simulink model "DAQTest"  (Simulink 7.9)
settings: Solver=FixedStepDiscrete  StartTime=0.0  StopTime=inf  FixedStep=0.001  RelTol=1e-3
undefined symbols (not defined in the file or in its folder): CalibrationParams, EncoderAngleLimits, EncoderThreshold, IMUAngleLimits, IMUThreshold, MotorParams
libraries: xpcethercatlib x160, simulink x3, marlo_lib_v01 x2, dspswit3 x1
(part 1 of 3)
settings Model: Creator=bgbuss  LastModifiedBy=bgbuss  BufferReuse=off
settings DataIOCC: LimitDataPoints=off
settings OptimizationCC: BlockReduction=off  OptimizeBlockIOStorage=off  BufferReuse=off  ExpressionFolding=off  LocalBlockOutputs=off
settings HardwareCC: ProdIntDivRoundTo=Zero  ProdEndianess=LittleEndian  ProdHWDeviceType=Generic->32-bit x86 compatible
settings RTWCC: SystemTargetFile=xpctarget.tlc  TemplateMakefile=xpc_default_tmf  Description=xPC Target  ProcessScript=xpctarget_make_rtw_hook  RTWCompilerOptimization=On
settings xpcTargetCC: TargetFcnLib=ansi_tfl_table_tmw.mat  CodeReplacementLibrary=XPC_BLAS  CodeExecutionProfiling=off  ParMdlRefBuildCompliant=on  ConcurrentExecutionCompliant=on  CombineSignalStateStructs=off  PortableWordSizes=off  GRTInterface=on  RL32LogBufSizeModifier=20000000  xPCTaskExecutionProfile=off  xPCRL32EventNumber=5000  xPCLoadParamSetFile=off  xPCConcurrentTasks=off  xPCEnableSFAnimation=off

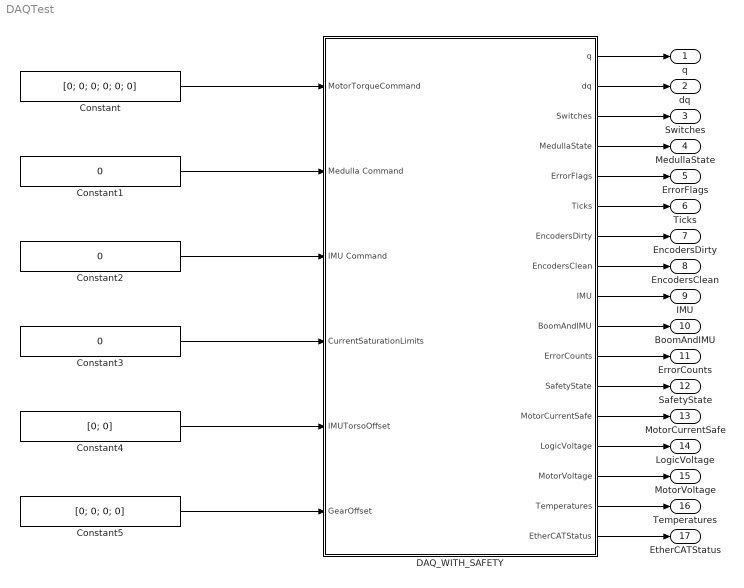
== system DAQTest ==
  Constant : Constant  Value=[0; 0; 0; 0; 0; 0]
  Constant1 : Constant  Value=0
  Constant2 : Constant  Value=0
  Constant3 : Constant  Value=0
  Constant4 : Constant  Value=[0; 0]
  Constant5 : Constant  Value=[0; 0; 0; 0]
  DAQ_WITH_SAFETY : Subsystem  AncestorBlock=marlo_lib_v01/DAQ_WITH_SAFETY
  q : Outport
  dq : Outport  Port=2
  Switches : Outport  Port=3
  MedullaState : Outport  Port=4
  ErrorFlags : Outport  Port=5
  Ticks : Outport  Port=6
  EncodersDirty : Outport  Port=7
  EncodersClean : Outport  Port=8
  IMU : Outport  Port=9
  BoomAndIMU : Outport  Port=10
  ErrorCounts : Outport  Port=11
  SafetyState : Outport  Port=12
  MotorCurrentSafe : Outport  Port=13
  LogicVoltage : Outport  Port=14
  MotorVoltage : Outport  Port=15
  Temperatures : Outport  Port=16
  EtherCATStatus : Outport  Port=17
  wires:
  DAQ_WITH_SAFETY/1(q) -> q/1
  DAQ_WITH_SAFETY/2(dq) -> dq/1
  DAQ_WITH_SAFETY/3(Switches) -> Switches/1
  DAQ_WITH_SAFETY/4(MedullaState) -> MedullaState/1
  DAQ_WITH_SAFETY/5(ErrorFlags) -> ErrorFlags/1
  DAQ_WITH_SAFETY/6(Ticks) -> Ticks/1
  DAQ_WITH_SAFETY/7(EncodersDirty) -> EncodersDirty/1
  DAQ_WITH_SAFETY/8(EncodersClean) -> EncodersClean/1
  DAQ_WITH_SAFETY/9(IMU) -> IMU/1
  DAQ_WITH_SAFETY/10(BoomAndIMU) -> BoomAndIMU/1
  DAQ_WITH_SAFETY/11(ErrorCounts) -> ErrorCounts/1
  DAQ_WITH_SAFETY/12(SafetyState) -> SafetyState/1
  DAQ_WITH_SAFETY/13(MotorCurrentSafe) -> MotorCurrentSafe/1
  Constant/1 -> DAQ_WITH_SAFETY/1(MotorTorqueCommand)
  Constant1/1 -> DAQ_WITH_SAFETY/2(Medulla Command)
  Constant2/1 -> DAQ_WITH_SAFETY/3(IMU Command)
  Constant3/1 -> DAQ_WITH_SAFETY/4(CurrentSaturationLimits)
  Constant4/1 -> DAQ_WITH_SAFETY/5(IMUTorsoOffset)
  Constant5/1 -> DAQ_WITH_SAFETY/6(GearOffset)
  DAQ_WITH_SAFETY/17(EtherCATStatus) -> EtherCATStatus/1
  DAQ_WITH_SAFETY/16(Temperatures) -> Temperatures/1
  DAQ_WITH_SAFETY/14(LogicVoltage) -> LogicVoltage/1
  DAQ_WITH_SAFETY/15(MotorVoltage) -> MotorVoltage/1

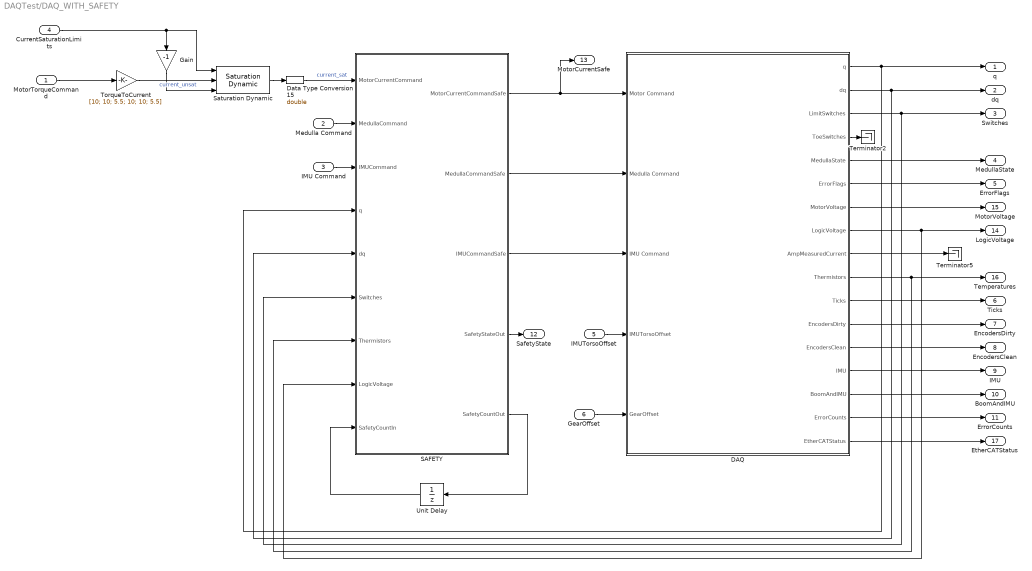
== system DAQTest/DAQ_WITH_SAFETY ==
  MotorTorqueCommand : Inport
  Medulla Command : Inport  Port=2
  IMU Command : Inport  Port=3
  CurrentSaturationLimits : Inport  Port=4
  IMUTorsoOffset : Inport  Port=5
  GearOffset : Inport  Port=6
  DAQ : Subsystem
  Data Type Conversion15 : DataTypeConversion  OutDataTypeStr=double
  Gain : Gain  Gain=-1
  SAFETY : MATLAB Function  TreatAsAtomicUnit=on
  Saturation Dynamic : simulink/Discontinuities/Saturation Dynamic  OutMin=[]  OutMax=[]  OutDataTypeStr=Inherit: Same as second input  OutDataType=fixdt(1, 16)  OutScaling=2^-10  DoSatur=off
  Terminator2 : Terminator
  Terminator5 : Terminator
  TorqueToCurrent : Gain  Gain=[10; 10; 5.5; 10; 10; 5.5]
  Unit Delay : UnitDelay  SampleTime=-1
  q : Outport
  dq : Outport  Port=2
  Switches : Outport  Port=3
  MedullaState : Outport  Port=4
  ErrorFlags : Outport  Port=5
  Ticks : Outport  Port=6
  EncodersDirty : Outport  Port=7
  EncodersClean : Outport  Port=8
  IMU : Outport  Port=9
  BoomAndIMU : Outport  Port=10
  ErrorCounts : Outport  Port=11
  SafetyState : Outport  Port=12
  MotorCurrentSafe : Outport  Port=13
  LogicVoltage : Outport  Port=14
  MotorVoltage : Outport  Port=15
  Temperatures : Outport  Port=16
  EtherCATStatus : Outport  Port=17
  wires:
  DAQ/13(EncodersClean) -> EncodersClean/1
  DAQ/16(ErrorCounts) -> ErrorCounts/1
  Unit Delay/1 -> SAFETY/9(SafetyCountIn)
  SAFETY/5(SafetyCountOut) -> Unit Delay/1
  GearOffset/1 -> DAQ/5(GearOffset)
  IMUTorsoOffset/1 -> DAQ/4(IMUTorsoOffset)
  DAQ/15(BoomAndIMU) -> BoomAndIMU/1
  Data Type Conversion15/1 -> SAFETY/1(MotorCurrentCommand)  "current_sat"
  SAFETY/2(MedullaCommandSafe) -> DAQ/2(Medulla Command)
  SAFETY/1(MotorCurrentCommandSafe) -> MotorCurrentSafe/1, DAQ/1(Motor Command)
  Gain/1 -> Saturation Dynamic/3
  CurrentSaturationLimits/1 -> Gain/1, Saturation Dynamic/1
  Saturation Dynamic/1 -> Data Type Conversion15/1
  DAQ/6(ErrorFlags) -> ErrorFlags/1
  DAQ/5(MedullaState) -> MedullaState/1
  DAQ/9(AmpMeasuredCurrent) -> Terminator5/1
  DAQ/7(MotorVoltage) -> MotorVoltage/1
  DAQ/10(Thermistors) -> SAFETY/7(Thermistors), Temperatures/1
  TorqueToCurrent/1 -> Saturation Dynamic/2  "current_unsat"
  SAFETY/4(SafetyStateOut) -> SafetyState/1
  DAQ/14(IMU) -> IMU/1
  DAQ/8(LogicVoltage) -> SAFETY/8(LogicVoltage), LogicVoltage/1
  DAQ/3(LimitSwitches) -> Switches/1, SAFETY/6(Switches)
  DAQ/2(dq) -> dq/1, SAFETY/5(dq)
  DAQ/1(q) -> q/1, SAFETY/4(q)
  IMU Command/1 -> SAFETY/3(IMUCommand)
  Medulla Command/1 -> SAFETY/2(MedullaCommand)
  MotorTorqueCommand/1 -> TorqueToCurrent/1
  SAFETY/3(IMUCommandSafe) -> DAQ/3(IMU Command)
  DAQ/11(Ticks) -> Ticks/1
  DAQ/12(EncodersDirty) -> EncodersDirty/1
  DAQ/4(ToeSwitches) -> Terminator2/1
  DAQ/17(EtherCATStatus) -> EtherCATStatus/1

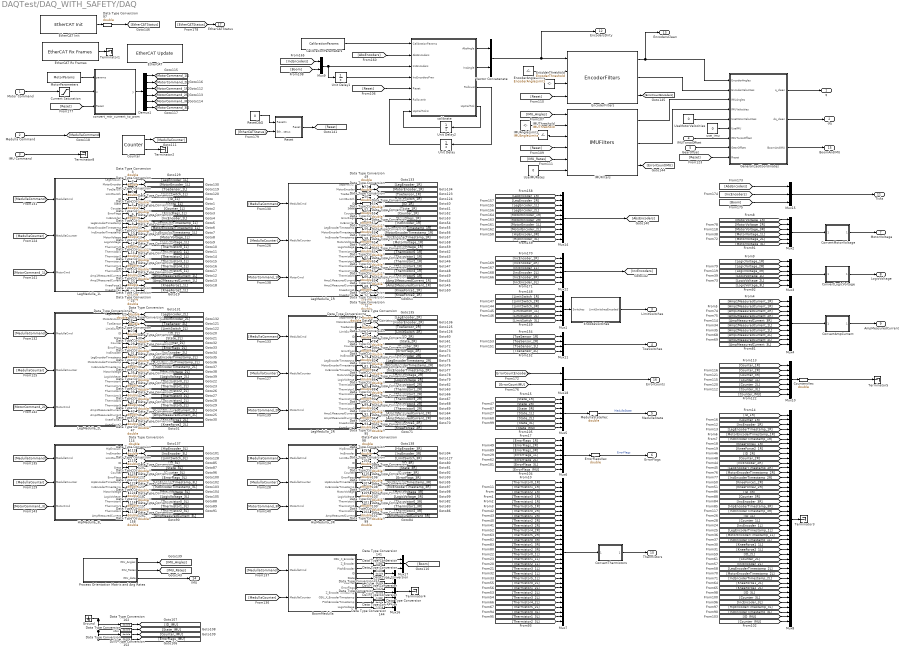
== system DAQTest/DAQ_WITH_SAFETY/DAQ ==
  Motor Command : Inport
  Medulla Command : Inport  Port=2
  IMU Command : Inport  Port=3
  IMUTorsoOffset : Inport  Port=4
  GearOffset : Inport  Port=5
  BoomMedulla : Subsystem
  CalibrationParameters : Constant  Value=CalibrationParams
  ConvertAmpCurrent : MATLAB Function  TreatAsAtomicUnit=on
  ConvertLogicVoltage : MATLAB Function  TreatAsAtomicUnit=on
  ConvertMotorVoltage : MATLAB Function  TreatAsAtomicUnit=on
  ConvertThermistors : MATLAB Function  TreatAsAtomicUnit=on
  Counter : dspswit3/Counter  Direction=Up  CountEvent=Free running  CounterSize=User defined  MaxCount=65535  InitialCount=0  Output=Count and Hit  HitValue=32  ResetInput=off  SamplesPerFrame=1  Ts=.001  CntDtype=double  HitDtype=Logical
  CountersVec : DataTypeConversion  OutDataTypeStr=double
  Current Saturation : Saturate  UpperLimit=50  LowerLimit=-50
  Data Type Conversion{1..112,114..126,131..133,138..145,152,154,157..158,161..162} (142 alike) : DataTypeConversion  OutDataTypeStr=double
  Demux1 : Demux  Outputs=6
  EncodeSwitches : MATLAB Function  TreatAsAtomicUnit=on
  EncoderAngleLimits : Constant  Value=EncoderAngleLimits
  EncoderFilters : marlo_lib_v01/EncoderFilters
  EncoderThreshold : Constant  Value=EncoderThreshold
  ErrorFlagsVec : DataTypeConversion  OutDataTypeStr=double
  EtherCAT : xpcethercatlib/EtherCAT Update   Priority=4  device_id=0  task_id_list=[1]  task_rates=[1]  task_priorities=[1500]
  EtherCAT Init : xpcethercatlib/EtherCAT Init   Priority=0  config_file='full_robot_eni_v4.xml'  device_id=0  pci_bus=5  pci_slot=5  enaDC=on  errRptLevel=0  sample_time=-1
  EtherCAT Rx Frames : xpcethercatlib/EtherCAT Rx Frames   Priority=1  device_id=0  sample_time=0
  GeneralizedCoordinates : MATLAB Function  TreatAsAtomicUnit=on
  Ground : Ground
  HipMedulla_3L : Subsystem
  HipMedulla_3R : Subsystem
  IMUAngleLimits : Constant  Value=IMUAngleLimits
  IMUFilters : marlo_lib_v01/IMUFilters
  IMUThreshold : Constant  Value=IMUThreshold
  LegMedulla_1L : Subsystem
  LegMedulla_1R : Subsystem
  LegMedulla_2L : Subsystem
  LegMedulla_2R : Subsystem
  MedullaStateVec : DataTypeConversion  OutDataTypeStr=double
  MotorParameters : Constant  Value=MotorParams
  Mux{1..3,12} (4 alike) : Mux  Inputs=6
  Mux10 : Mux  Inputs=7
  Mux11 : Mux
  Mux14 : Mux  Inputs=10
  Mux15 : Mux  Inputs=3
  Mux16 : Mux  Inputs=8
  Mux17 : Mux  Inputs=3
  Mux18 : Mux  Inputs=2
  Mux4 : Mux  Inputs=10
  Mux5 : Mux  Inputs=7
  Mux6 : Mux  Inputs=7
  Mux7 : Mux  Inputs=30
  Mux8 : Mux  Inputs=44
  Mux9 : Mux  Inputs=2
  Process Orientation Matrix and Ang Rates : Subsystem
  Reset : Subsystem
  ResetDAQ : Constant  Value=0
  Terminator{1..5,8} (6 alike) : Terminator
  Unit Delay : UnitDelay  X0=zeros(9,1)  SampleTime=-1
  Unit Delay1 : UnitDelay  SampleTime=-1
  Unit Delay2 : UnitDelay  X0=zeros(2,1)  SampleTime=-1
  UseIMURates : Constant  Value=0
  UseMotorVelocities : Constant  Value=0
  Vector Concatenate : Concatenate
  calibrate : MATLAB Function  TreatAsAtomicUnit=on
  convert_mtr_current_to_pwm : MATLAB Function  TreatAsAtomicUnit=on
  use_imu : Constant  Value=0
  q : Outport
  dq : Outport  Port=2
  LimitSwitches : Outport  Port=3
  ToeSwitches : Outport  Port=4
  MedullaState : Outport  Port=5
  ErrorFlags : Outport  Port=6
  MotorVoltage : Outport  Port=7
  LogicVoltage : Outport  Port=8
  AmpMeasuredCurrent : Outport  Port=9
  Thermistors : Outport  Port=10
  Ticks : Outport  Port=11
  EncodersDirty : Outport  Port=12
  EncodersClean : Outport  Port=13
  IMU : Outport  Port=14
  BoomAndIMU : Outport  Port=15
  ErrorCounts : Outport  Port=16
  EtherCATStatus : Outport  Port=17
  wires:
  [ErrorCountIMU] -> Mux18/2
  [ErrorCountEncoders] -> Mux18/1
  Mux18/1 -> ErrorCounts/1
  IMUFilters/3 -> [ErrorCountIMU]
  EncoderFilters/3 -> [ErrorCountEncoders]
  EncoderFilters/1 -> EncodersClean/1, GeneralizedCoordinates/1(EncoderAngles)
  EncoderFilters/2 -> GeneralizedCoordinates/2(EncoderVelocities)
  IMUFilters/1 -> GeneralizedCoordinates/3(IMUAngles)
  IMUFilters/2 -> GeneralizedCoordinates/4(IMUVelocities)
  UseMotorVelocities/1 -> GeneralizedCoordinates/5(UseMotorVelocities)
  [Reset] -> GeneralizedCoordinates/9(Reset)
  GearOffset/1 -> GeneralizedCoordinates/8(GearOffset)
  IMUTorsoOffset/1 -> GeneralizedCoordinates/7(IMUTorsoOffset)
  IMUAngleLimits/1 -> IMUFilters/2
  IMUThreshold/1 -> IMUFilters/3
  EncoderThreshold/1 -> EncoderFilters/3
  EncoderAngleLimits/1 -> EncoderFilters/2
  Vector Concatenate/1 -> EncodersDirty/1, EncoderFilters/1
  calibrate/2(IncAngle) -> Vector Concatenate/2
  calibrate/1(AbsAngle) -> Vector Concatenate/1
  [IMU_Rates] -> IMUFilters/5
  UseIMURates/1 -> IMUFilters/6
  [Reset] -> IMUFilters/4
  [Reset] -> EncoderFilters/4
  [IMU_Angles] -> IMUFilters/1
  calibrate/4(HipCalTick) -> Unit Delay2/1
  Unit Delay2/1 -> calibrate/7(HipCalTickIn)
  Mux9/1 -> Unit Delay1/1, calibrate/3(IncEncoders)
  [Boom] -> Mux9/2
  [IncEncoders] -> Mux9/1
  Unit Delay1/1 -> calibrate/4(IncEncodersPrev)
  ResetDAQ/1 -> Reset/1(ResetIn)
  Reset/1(Reset) -> [Reset]
  [Reset] -> calibrate/5(Reset)
  [HipEncoder_3L] -> Mux14/10
  [HipEncoder_3R] -> Mux14/9
  [MotorEncoder_2L] -> Mux14/8
  [MotorEncoder_1L] -> Mux14/7
  [MotorEncoder_2R] -> Mux14/6
  [MotorEncoder_1R] -> Mux14/5
  Unit Delay/1 -> calibrate/6(RolloverIn)
  calibrate/3(Rollover) -> Unit Delay/1
  [AbsEncoders] -> calibrate/2(AbsEncoders)
  IMU Command/1 -> Terminator8/1
  [Boom] -> Mux15/3
  [IncEncoders] -> Mux15/2
  [AbsEncoders] -> Mux15/1
  Mux14/1 -> [AbsEncoders]
  Mux12/1 -> [IncEncoders]
  [LegEncoder_2L] -> Mux14/4
  [LegEncoder_1L] -> Mux14/3
  [LegEncoder_2R] -> Mux14/2
  [LegEncoder_1R] -> Mux14/1
  [IncEncoder_3L] -> Mux12/6
  [IncEncoder_2L] -> Mux12/4
  [IncEncoder_1L] -> Mux12/3
  [IncEncoder_3R] -> Mux12/5
  [IncEncoder_2R] -> Mux12/2
  [IncEncoder_1R] -> Mux12/1
  Data Type Conversion74/1 -> [MotorEncoder_2R]
  Data Type Conversion73/1 -> [LegEncoder_2R]
  Data Type Conversion50/1 -> [MotorEncoder_1R]
  Data Type Conversion49/1 -> [LegEncoder_1R]
  Data Type Conversion26/1 -> [MotorEncoder_2L]
  Data Type Conversion25/1 -> [LegEncoder_2L]
  Data Type Conversion1/1 -> [MotorEncoder_1L]
  Data Type Conversion3/1 -> [LegEncoder_1L]
  Process Orientation Matrix and Ang Rates/1(IMU_Angles) -> [IMU_Angles]
  Data Type Conversion4/1 -> [LimitSwitch_1L]
  Data Type Conversion2/1 -> [ToeSensor_1L]
  Data Type Conversion28/1 -> [LimitSwitch_2L]
  Data Type Conversion27/1 -> [ToeSensor_2L]
  Data Type Conversion52/1 -> [LimitSwitch_1R]
  Data Type Conversion51/1 -> [ToeSensor_1R]
  Data Type Conversion75/1 -> [ToeSensor_2R]
  Data Type Conversion76/1 -> [LimitSwitch_2R]
  [ToeSensor_2L] -> Mux11/4
  [ToeSensor_1L] -> Mux11/3
  [ToeSensor_2R] -> Mux11/2
  [ToeSensor_1R] -> Mux11/1
  [LimitSwitch_3L] -> Mux1/6
  [LimitSwitch_2L] -> Mux1/5
  [LimitSwitch_1L] -> Mux1/4
  [LimitSwitch_3R] -> Mux1/3
  [LimitSwitch_2R] -> Mux1/2
  [LimitSwitch_1R] -> Mux1/1
  Data Type Conversion112/1 -> [LimitSwitch_3L]
  Data Type Conversion157/1 -> [LimitSwitch_3R]
  Demux1/5 -> [MotorCommand_3R]
  Demux1/4 -> [MotorCommand_2R]
  Demux1/3 -> [MotorCommand_1R]
  Demux1/2 -> [MotorCommand_2L]
  Demux1/1 -> [MotorCommand_1L]
  [MotorCommand_3L] -> HipMedulla_3L/3(MotorCmd)
  Demux1/6 -> [MotorCommand_3L]
  [MotorCommand_3R] -> HipMedulla_3R/3(MotorCmd)
  [MotorCommand_2R] -> LegMedulla_2R/3(MotorCmd)
  [MotorCommand_1R] -> LegMedulla_1R/3(MotorCmd)
  [MotorCommand_2L] -> LegMedulla_2L/3(MotorCmd)
  [MotorCommand_1L] -> LegMedulla_1L/3(MotorCmd)
  [MedullaCounter] -> BoomMedulla/2(MedullaCounter)
  [MedullaCommand] -> BoomMedulla/1(MedullaCmd)
  [MedullaCommand] -> HipMedulla_3L/1(MedullaCmd)
  [MedullaCommand] -> HipMedulla_3R/1(MedullaCmd)
  [MedullaCommand] -> LegMedulla_1L/1(MedullaCmd)
  [MedullaCommand] -> LegMedulla_2L/1(MedullaCmd)
  [MedullaCommand] -> LegMedulla_2R/1(MedullaCmd)
  [MedullaCommand] -> LegMedulla_1R/1(MedullaCmd)
  [MedullaCounter] -> LegMedulla_2L/2(MedullaCounter)
  [MedullaCounter] -> LegMedulla_1R/2(MedullaCounter)
  [MedullaCounter] -> LegMedulla_2R/2(MedullaCounter)
  [MedullaCounter] -> HipMedulla_3R/2(MedullaCounter)
  [MedullaCounter] -> HipMedulla_3L/2(MedullaCounter)
  [MedullaCounter] -> LegMedulla_1L/2(MedullaCounter)
  Counter/1 -> [MedullaCounter]
  Mux16/1 -> Terminator4/1
  BoomMedulla/11(LogicVoltage) -> Data Type Conversion144/1
  BoomMedulla/10(PitchEncoderTimestamp) -> Data Type Conversion145/1
  BoomMedulla/9(OSU_X_EncoderTimestamp) -> Data Type Conversion131/1
  BoomMedulla/8(Z_EncoderTimestamp) -> Data Type Conversion133/1
  BoomMedulla/7(ErrorFlags) -> Data Type Conversion138/1
  BoomMedulla/6(Counter) -> Data Type Conversion132/1
  BoomMedulla/5(State) -> Data Type Conversion142/1
  BoomMedulla/4(ID) -> Data Type Conversion143/1
  BoomMedulla/3(PitchEncoder) -> Data Type Conversion139/1
  Data Type Conversion141/1 -> Mux17/1
  Data Type Conversion140/1 -> Mux17/2
  Data Type Conversion139/1 -> Mux17/3
  Data Type Conversion143/1 -> Mux16/1
  Data Type Conversion142/1 -> Mux16/2
  Data Type Conversion132/1 -> Mux16/3
  Data Type Conversion138/1 -> Mux16/4
  Data Type Conversion133/1 -> Mux16/5
  Data Type Conversion131/1 -> Mux16/6
  Data Type Conversion145/1 -> Mux16/7
  Data Type Conversion144/1 -> Mux16/8
  Process Orientation Matrix and Ang Rates/2(IMU_Rates) -> [IMU_Rates]
  GeneralizedCoordinates/3(BoomAndIMU) -> BoomAndIMU/1
  GeneralizedCoordinates/2(dq_clean) -> dq/1
  GeneralizedCoordinates/1(q_clean) -> q/1
  use_imu/1 -> GeneralizedCoordinates/6(UseIMU)
  Mux17/1 -> [Boom]
  [Counter_IMU] -> Mux10/7
  [Counter_3L] -> Mux10/6
  [Counter_2L] -> Mux10/5
  [Counter_1L] -> Mux10/4
  [Counter_3R] -> Mux10/3
  [Counter_2R] -> Mux10/2
  [Counter_1R] -> Mux10/1
  Mux10/1 -> CountersVec/1
  CountersVec/1 -> Terminator5/1
  ErrorFlagsVec/1 -> ErrorFlags/1  "ErrorFlags"
  MedullaStateVec/1 -> MedullaState/1  "MedullaState"
  ConvertAmpCurrent/1(measuredCurrent) -> AmpMeasuredCurrent/1
  ConvertThermistors/1(temperature) -> Thermistors/1
  ConvertLogicVoltage/1(logicVoltage) -> LogicVoltage/1
  ConvertMotorVoltage/1(motorVoltage) -> MotorVoltage/1
  Mux6/1 -> ErrorFlagsVec/1
  Mux5/1 -> MedullaStateVec/1
  Mux4/1 -> ConvertAmpCurrent/1(adc_value)
  Mux3/1 -> ConvertLogicVoltage/1(adc_value)
  Mux2/1 -> ConvertMotorVoltage/1(adc_value)
  [State_IMU] -> Mux5/7
  [ErrorFlags_IMU] -> Mux6/7
  [Counter_IMU] -> Mux8/44
  [ID_IMU] -> Mux8/43
  Data Type Conversion154/1 -> [ErrorFlags_IMU]
  Data Type Conversion152/1 -> [Counter_IMU]
  Data Type Conversion161/1 -> [State_IMU]
  Data Type Conversion162/1 -> [ID_IMU]
  Mux8/1 -> Terminator3/1
  [IncEncoderTimestamp_3L] -> Mux8/42
  [HipEncoderTimestamp_3L] -> Mux8/41
  [IncEncoder_3L] -> Mux8/40
  [Counter_3L] -> Mux8/39
  [ID_3L] -> Mux8/38
  [KneeForce2_2L] -> Mux8/37
  [KneeForce1_2L] -> Mux8/36
  [IncEncoderTimestamp_2L] -> Mux8/35
  [MotorEncoderTimestamp_2L] -> Mux8/34
  [LegEncoderTimestamp_2L] -> Mux8/33
  [IncEncoder_2L] -> Mux8/32
  [Counter_2L] -> Mux8/31
  [ID_2L] -> Mux8/30
  [KneeForce2_1L] -> Mux8/29
  [KneeForce1_1L] -> Mux8/28
  [IncEncoderTimestamp_1L] -> Mux8/27
  [MotorEncoderTimestamp_1L] -> Mux8/26
  [LegEncoderTimestamp_1L] -> Mux8/25
  [IncEncoder_1L] -> Mux8/24
  [Counter_1L] -> Mux8/23
  [ID_1L] -> Mux8/22
  [IncEncoderTimestamp_3R] -> Mux8/21
  [HipEncoderTimestamp_3R] -> Mux8/20
  [IncEncoder_3R] -> Mux8/19
  [Counter_3R] -> Mux8/18
  [ID_3R] -> Mux8/17
  [KneeForce2_2R] -> Mux8/16
  [KneeForce1_2R] -> Mux8/15
  [IncEncoderTimestamp_2R] -> Mux8/14
  [MotorEncoderTimestamp_2R] -> Mux8/13
  [LegEncoderTimestamp_2R] -> Mux8/12
  [IncEncoder_2R] -> Mux8/11
  [Counter_2R] -> Mux8/10
  [ID_2R] -> Mux8/9
  [KneeForce2_1R] -> Mux8/8
  [KneeForce1_1R] -> Mux8/7
  [IncEncoderTimestamp_1R] -> Mux8/6
  [MotorEncoderTimestamp_1R] -> Mux8/5
  [LegEncoderTimestamp_1R] -> Mux8/4
  [IncEncoder_1R] -> Mux8/3
  [Counter_1R] -> Mux8/2
  [ID_1R] -> Mux8/1
  [ErrorFlags_3L] -> Mux6/6
  [ErrorFlags_2L] -> Mux6/5
  [ErrorFlags_1L] -> Mux6/4
  [ErrorFlags_3R] -> Mux6/3
  [ErrorFlags_2R] -> Mux6/2
  [ErrorFlags_1R] -> Mux6/1
  [State_3L] -> Mux5/6
  [State_2L] -> Mux5/5
  [State_1L] -> Mux5/4
  [State_3R] -> Mux5/3
  [State_2R] -> Mux5/2
  [State_1R] -> Mux5/1
  [AmpMeasuredCurrent_3L] -> Mux4/10
  [Amp2MeasuredCurrent_2L] -> Mux4/9
  [Amp1MeasuredCurrent_2L] -> Mux4/8
  [Amp2MeasuredCurrent_1L] -> Mux4/7
  [Amp1MeasuredCurrent_1L] -> Mux4/6
  [AmpMeasuredCurrent_3R] -> Mux4/5
  [Amp2MeasuredCurrent_2R] -> Mux4/4
  [Amp1MeasuredCurrent_2R] -> Mux4/3
  [Amp2MeasuredCurrent_1R] -> Mux4/2
  [Amp1MeasuredCurrent_1R] -> Mux4/1
  [LogicVoltage_3L] -> Mux3/6
  [LogicVoltage_2L] -> Mux3/5
  [LogicVoltage_1L] -> Mux3/4
  [LogicVoltage_3R] -> Mux3/3
  [LogicVoltage_2R] -> Mux3/2
  [LogicVoltage_1R] -> Mux3/1
  [MotorVoltage_3L] -> Mux2/6
  [MotorVoltage_2L] -> Mux2/5
  [MotorVoltage_1L] -> Mux2/4
  [MotorVoltage_3R] -> Mux2/3
  [MotorVoltage_2R] -> Mux2/2
  [MotorVoltage_1R] -> Mux2/1
  Mux7/1 -> ConvertThermistors/1(adc_value)
  [Thermistor2_3L] -> Mux7/30
  [Thermistor1_3L] -> Mux7/29
  [Thermistor0_3L] -> Mux7/28
  [Thermistor5_2L] -> Mux7/27
  [Thermistor4_2L] -> Mux7/26
  [Thermistor3_2L] -> Mux7/25
  [Thermistor2_2L] -> Mux7/24
  [Thermistor1_2L] -> Mux7/23
  [Thermistor0_2L] -> Mux7/22
  [Thermistor5_1L] -> Mux7/21
  [Thermistor4_1L] -> Mux7/20
  [Thermistor3_1L] -> Mux7/19
  [Thermistor2_1L] -> Mux7/18
  [Thermistor1_1L] -> Mux7/17
  [Thermistor0_1L] -> Mux7/16
  [Thermistor2_3R] -> Mux7/15
  [Thermistor1_3R] -> Mux7/14
  [Thermistor0_3R] -> Mux7/13
  [Thermistor5_2R] -> Mux7/12
  [Thermistor4_2R] -> Mux7/11
  [Thermistor3_2R] -> Mux7/10
  [Thermistor2_2R] -> Mux7/9
  [Thermistor1_2R] -> Mux7/8
  [Thermistor0_2R] -> Mux7/7
  [Thermistor5_1R] -> Mux7/6
  [Thermistor4_1R] -> Mux7/5
  [Thermistor3_1R] -> Mux7/4
  [Thermistor2_1R] -> Mux7/3
  [Thermistor1_1R] -> Mux7/2
  [Thermistor0_1R] -> Mux7/1
  Data Type Conversion24/1 -> [KneeForce2_1L]
  Data Type Conversion23/1 -> [KneeForce1_1L]
  Data Type Conversion22/1 -> [Amp2MeasuredCurrent_1L]
  Data Type Conversion21/1 -> [Amp1MeasuredCurrent_1L]
  Data Type Conversion20/1 -> [Thermistor5_1L]
  Data Type Conversion19/1 -> [Thermistor4_1L]
  Data Type Conversion18/1 -> [Thermistor3_1L]
  Data Type Conversion17/1 -> [Thermistor2_1L]
  Data Type Conversion16/1 -> [Thermistor1_1L]
  Data Type Conversion15/1 -> [Thermistor0_1L]
  Data Type Conversion14/1 -> [LogicVoltage_1L]
  Data Type Conversion13/1 -> [MotorVoltage_1L]
  Data Type Conversion12/1 -> [IncEncoderTimestamp_1L]
  Data Type Conversion11/1 -> [MotorEncoderTimestamp_1L]
  Data Type Conversion10/1 -> [LegEncoderTimestamp_1L]
  Data Type Conversion9/1 -> [IncEncoder_1L]
  Data Type Conversion8/1 -> [ErrorFlags_1L]
  Ground/1 -> Data Type Conversion162/1, Data Type Conversion161/1, Data Type Conversion152/1, Data Type Conversion154/1
  Process Orientation Matrix and Ang Rates/3(IMU_data) -> IMU/1
  CalibrationParameters/1 -> calibrate/1(CalibrationParams)
  Mux15/1 -> Ticks/1
  Mux1/1 -> EncodeSwitches/1(Switches)
  HipMedulla_3L/15(AmpMeasuredCurrent) -> Data Type Conversion126/1
  HipMedulla_3L/14(Thermistor2) -> Data Type Conversion158/1
  HipMedulla_3L/13(Thermistor1) -> Data Type Conversion115/1
  HipMedulla_3L/12(Thermistor0) -> Data Type Conversion117/1
  HipMedulla_3L/11(LogicVoltage) -> Data Type Conversion118/1
  HipMedulla_3L/10(MotorVoltage) -> Data Type Conversion116/1
  HipMedulla_3L/9(IncEncoderTimestamp) -> Data Type Conversion123/1
  HipMedulla_3L/8(HipEncoderTimestamp) -> Data Type Conversion124/1
  HipMedulla_3L/7(ErrorFlags) -> Data Type Conversion121/1
  HipMedulla_3L/6(Counter) -> Data Type Conversion122/1
  HipMedulla_3L/5(State) -> Data Type Conversion120/1
  HipMedulla_3L/4(ID) -> Data Type Conversion125/1
  Data Type Conversion125/1 -> [ID_3L]
  Data Type Conversion120/1 -> [State_3L]
  Data Type Conversion122/1 -> [Counter_3L]
  Data Type Conversion121/1 -> [ErrorFlags_3L]
  Data Type Conversion119/1 -> [IncEncoder_3L]
  Data Type Conversion124/1 -> [HipEncoderTimestamp_3L]
  Data Type Conversion123/1 -> [IncEncoderTimestamp_3L]
  Data Type Conversion116/1 -> [MotorVoltage_3L]
  Data Type Conversion118/1 -> [LogicVoltage_3L]
  Data Type Conversion117/1 -> [Thermistor0_3L]
  Data Type Conversion115/1 -> [Thermistor1_3L]
  Data Type Conversion158/1 -> [Thermistor2_3L]
  Data Type Conversion126/1 -> [AmpMeasuredCurrent_3L]
  HipMedulla_3L/2(IncEncoder) -> Data Type Conversion119/1
  HipMedulla_3L/1(HipEncoder) -> Data Type Conversion114/1
  Data Type Conversion114/1 -> [HipEncoder_3L]
  HipMedulla_3L/3(LimitSwitch) -> Data Type Conversion112/1
  HipMedulla_3R/15(AmpMeasuredCurrent) -> Data Type Conversion111/1
  HipMedulla_3R/14(Thermistor2) -> Data Type Conversion99/1
  HipMedulla_3R/13(Thermistor1) -> Data Type Conversion100/1
  HipMedulla_3R/12(Thermistor0) -> Data Type Conversion102/1
  HipMedulla_3R/11(LogicVoltage) -> Data Type Conversion103/1
  HipMedulla_3R/10(MotorVoltage) -> Data Type Conversion101/1
  HipMedulla_3R/9(IncEncoderTimestamp) -> Data Type Conversion108/1
  HipMedulla_3R/8(HipEncoderTimestamp) -> Data Type Conversion109/1
  HipMedulla_3R/7(ErrorFlags) -> Data Type Conversion106/1
  HipMedulla_3R/6(Counter) -> Data Type Conversion107/1
  HipMedulla_3R/5(State) -> Data Type Conversion105/1
  HipMedulla_3R/4(ID) -> Data Type Conversion110/1
  HipMedulla_3R/3(LimitSwitch) -> Data Type Conversion157/1
  HipMedulla_3R/2(IncEncoder) -> Data Type Conversion104/1
  HipMedulla_3R/1(HipEncoder) -> Data Type Conversion98/1
  Data Type Conversion98/1 -> [HipEncoder_3R]
  Data Type Conversion110/1 -> [ID_3R]
  Data Type Conversion105/1 -> [State_3R]
  Data Type Conversion107/1 -> [Counter_3R]
  Data Type Conversion106/1 -> [ErrorFlags_3R]
  Data Type Conversion104/1 -> [IncEncoder_3R]
  Data Type Conversion109/1 -> [HipEncoderTimestamp_3R]
  Data Type Conversion108/1 -> [IncEncoderTimestamp_3R]
  Data Type Conversion101/1 -> [MotorVoltage_3R]
  Data Type Conversion103/1 -> [LogicVoltage_3R]
  Data Type Conversion102/1 -> [Thermistor0_3R]
  Data Type Conversion100/1 -> [Thermistor1_3R]
  Data Type Conversion99/1 -> [Thermistor2_3R]
  convert_mtr_current_to_pwm/1(y) -> Demux1/1
  Data Type Conversion48/1 -> [KneeForce2_2L]
  Data Type Conversion47/1 -> [KneeForce1_2L]
  Data Type Conversion46/1 -> [Amp2MeasuredCurrent_2L]
  Data Type Conversion45/1 -> [Amp1MeasuredCurrent_2L]
  Data Type Conversion44/1 -> [Thermistor5_2L]
  Data Type Conversion43/1 -> [Thermistor4_2L]
  Data Type Conversion42/1 -> [Thermistor3_2L]
  Data Type Conversion41/1 -> [Thermistor2_2L]
  Data Type Conversion40/1 -> [Thermistor1_2L]
  Data Type Conversion39/1 -> [Thermistor0_2L]
  Data Type Conversion38/1 -> [LogicVoltage_2L]
  Data Type Conversion37/1 -> [MotorVoltage_2L]
  Data Type Conversion36/1 -> [IncEncoderTimestamp_2L]
  Data Type Conversion35/1 -> [MotorEncoderTimestamp_2L]
  Data Type Conversion34/1 -> [LegEncoderTimestamp_2L]
  Data Type Conversion33/1 -> [IncEncoder_2L]
  Data Type Conversion32/1 -> [ErrorFlags_2L]
  Data Type Conversion31/1 -> [Counter_2L]
  Data Type Conversion30/1 -> [State_2L]
  Data Type Conversion29/1 -> [ID_2L]
  Data Type Conversion7/1 -> [Counter_1L]
  Data Type Conversion6/1 -> [State_1L]
  Data Type Conversion5/1 -> [ID_1L]
  LegMedulla_1R/1(LegEncoder) -> Data Type Conversion49/1
  LegMedulla_1L/1(LegEncoder) -> Data Type Conversion3/1
  LegMedulla_1R/2(MotorEncoder) -> Data Type Conversion50/1
  Current Saturation/1 -> convert_mtr_current_to_pwm/2(u)
  MotorParameters/1 -> convert_mtr_current_to_pwm/1(params)
  Motor Command/1 -> Current Saturation/1
  Data Type Conversion111/1 -> [AmpMeasuredCurrent_3R]
  Data Type Conversion96/1 -> [KneeForce2_2R]
  Data Type Conversion95/1 -> [KneeForce1_2R]
  Data Type Conversion94/1 -> [Amp2MeasuredCurrent_2R]
  Data Type Conversion93/1 -> [Amp1MeasuredCurrent_2R]
  Data Type Conversion92/1 -> [Thermistor5_2R]
  Data Type Conversion91/1 -> [Thermistor4_2R]
  Data Type Conversion90/1 -> [Thermistor3_2R]
  Data Type Conversion89/1 -> [Thermistor2_2R]
  Data Type Conversion88/1 -> [Thermistor1_2R]
  Data Type Conversion87/1 -> [Thermistor0_2R]
  Data Type Conversion86/1 -> [LogicVoltage_2R]
  Data Type Conversion85/1 -> [MotorVoltage_2R]
  Data Type Conversion84/1 -> [IncEncoderTimestamp_2R]
  Data Type Conversion83/1 -> [MotorEncoderTimestamp_2R]
  Data Type Conversion82/1 -> [LegEncoderTimestamp_2R]
  Data Type Conversion81/1 -> [IncEncoder_2R]
  Data Type Conversion80/1 -> [ErrorFlags_2R]
  Data Type Conversion79/1 -> [Counter_2R]
  Data Type Conversion78/1 -> [State_2R]
  Data Type Conversion77/1 -> [ID_2R]
  Data Type Conversion72/1 -> [KneeForce2_1R]
  Data Type Conversion71/1 -> [KneeForce1_1R]
  Data Type Conversion70/1 -> [Amp2MeasuredCurrent_1R]
  Data Type Conversion69/1 -> [Amp1MeasuredCurrent_1R]
  Data Type Conversion68/1 -> [Thermistor5_1R]
  Data Type Conversion67/1 -> [Thermistor4_1R]
  Data Type Conversion66/1 -> [Thermistor3_1R]
  Data Type Conversion65/1 -> [Thermistor2_1R]
  Data Type Conversion64/1 -> [Thermistor1_1R]
  Data Type Conversion63/1 -> [Thermistor0_1R]
  Data Type Conversion62/1 -> [LogicVoltage_1R]
  Data Type Conversion61/1 -> [MotorVoltage_1R]
  Data Type Conversion60/1 -> [IncEncoderTimestamp_1R]
  Data Type Conversion59/1 -> [MotorEncoderTimestamp_1R]
  Data Type Conversion58/1 -> [LegEncoderTimestamp_1R]
  Data Type Conversion57/1 -> [IncEncoder_1R]
  Data Type Conversion56/1 -> [ErrorFlags_1R]
  Data Type Conversion55/1 -> [Counter_1R]
  Data Type Conversion54/1 -> [State_1R]
  Data Type Conversion53/1 -> [ID_1R]
  LegMedulla_2R/3(ToeSensor) -> Data Type Conversion75/1
  LegMedulla_2R/2(MotorEncoder) -> Data Type Conversion74/1
  LegMedulla_2R/1(LegEncoder) -> Data Type Conversion73/1
  Counter/2 -> Terminator2/1
  EtherCAT Rx Frames/1 -> Terminator1/1
  Medulla Command/1 -> [MedullaCommand]
  LegMedulla_2R/24(KneeForce2) -> Data Type Conversion96/1
  LegMedulla_1R/24(KneeForce2) -> Data Type Conversion72/1
  LegMedulla_2R/23(KneeForce1) -> Data Type Conversion95/1
  LegMedulla_2R/22(Amp2MeasuredCurrent) -> Data Type Conversion94/1
  LegMedulla_2R/21(Amp1MeasuredCurrent) -> Data Type Conversion93/1
  LegMedulla_2R/20(Thermistor5) -> Data Type Conversion92/1
  LegMedulla_2R/19(Thermistor4) -> Data Type Conversion91/1
  LegMedulla_2R/18(Thermistor3) -> Data Type Conversion90/1
  LegMedulla_2R/17(Thermistor2) -> Data Type Conversion89/1
  LegMedulla_2R/16(Thermistor1) -> Data Type Conversion88/1
  LegMedulla_2R/15(Thermistor0) -> Data Type Conversion87/1
  LegMedulla_2R/14(LogicVoltage) -> Data Type Conversion86/1
  LegMedulla_2R/13(MotorVoltage) -> Data Type Conversion85/1
  LegMedulla_2R/12(IncEncoderTimestamp) -> Data Type Conversion84/1
  LegMedulla_2R/11(MotorEncoderTimestamp) -> Data Type Conversion83/1
  LegMedulla_2R/10(LegEncoderTimestamp) -> Data Type Conversion82/1
  LegMedulla_2R/9(IncEncoder) -> Data Type Conversion81/1
  LegMedulla_2R/8(ErrorFlags) -> Data Type Conversion80/1
  LegMedulla_2R/7(Counter) -> Data Type Conversion79/1
  LegMedulla_2R/6(State) -> Data Type Conversion78/1
  LegMedulla_2R/5(ID) -> Data Type Conversion77/1
  LegMedulla_2R/4(LimitSwitch) -> Data Type Conversion76/1
  LegMedulla_1R/23(KneeForce1) -> Data Type Conversion71/1
  LegMedulla_1R/22(Amp2MeasuredCurrent) -> Data Type Conversion70/1
  LegMedulla_1R/21(Amp1MeasuredCurrent) -> Data Type Conversion69/1
  LegMedulla_1R/20(Thermistor5) -> Data Type Conversion68/1
  LegMedulla_1R/19(Thermistor4) -> Data Type Conversion67/1
  LegMedulla_1R/18(Thermistor3) -> Data Type Conversion66/1
  LegMedulla_1R/17(Thermistor2) -> Data Type Conversion65/1
  LegMedulla_1R/16(Thermistor1) -> Data Type Conversion64/1
  LegMedulla_1R/15(Thermistor0) -> Data Type Conversion63/1
  LegMedulla_1R/14(LogicVoltage) -> Data Type Conversion62/1
  LegMedulla_1R/13(MotorVoltage) -> Data Type Conversion61/1
  LegMedulla_1R/12(IncEncoderTimestamp) -> Data Type Conversion60/1
  LegMedulla_1R/11(MotorEncoderTimestamp) -> Data Type Conversion59/1
  LegMedulla_1R/10(LegEncoderTimestamp) -> Data Type Conversion58/1
  LegMedulla_1R/9(IncEncoder) -> Data Type Conversion57/1
  LegMedulla_1R/8(ErrorFlags) -> Data Type Conversion56/1
  LegMedulla_1R/7(Counter) -> Data Type Conversion55/1
  LegMedulla_1R/6(State) -> Data Type Conversion54/1
  LegMedulla_1R/5(ID) -> Data Type Conversion53/1
  LegMedulla_1R/4(LimitSwitch) -> Data Type Conversion52/1
  LegMedulla_1R/3(ToeSensor) -> Data Type Conversion51/1
  LegMedulla_2L/24(KneeForce2) -> Data Type Conversion48/1
  LegMedulla_1L/24(KneeForce2) -> Data Type Conversion24/1
  LegMedulla_2L/23(KneeForce1) -> Data Type Conversion47/1
  LegMedulla_2L/22(Amp2MeasuredCurrent) -> Data Type Conversion46/1
  LegMedulla_2L/21(Amp1MeasuredCurrent) -> Data Type Conversion45/1
  LegMedulla_2L/20(Thermistor5) -> Data Type Conversion44/1
  LegMedulla_2L/19(Thermistor4) -> Data Type Conversion43/1
  LegMedulla_2L/18(Thermistor3) -> Data Type Conversion42/1
  LegMedulla_2L/17(Thermistor2) -> Data Type Conversion41/1
  LegMedulla_2L/16(Thermistor1) -> Data Type Conversion40/1
  LegMedulla_2L/15(Thermistor0) -> Data Type Conversion39/1
  LegMedulla_2L/14(LogicVoltage) -> Data Type Conversion38/1
  LegMedulla_2L/13(MotorVoltage) -> Data Type Conversion37/1
  LegMedulla_2L/12(IncEncoderTimestamp) -> Data Type Conversion36/1
  LegMedulla_2L/11(MotorEncoderTimestamp) -> Data Type Conversion35/1
  LegMedulla_2L/10(LegEncoderTimestamp) -> Data Type Conversion34/1
  LegMedulla_2L/9(IncEncoder) -> Data Type Conversion33/1
  LegMedulla_2L/8(ErrorFlags) -> Data Type Conversion32/1
  LegMedulla_2L/7(Counter) -> Data Type Conversion31/1
  LegMedulla_2L/6(State) -> Data Type Conversion30/1
  LegMedulla_2L/5(ID) -> Data Type Conversion29/1
  LegMedulla_2L/4(LimitSwitch) -> Data Type Conversion28/1
  LegMedulla_2L/3(ToeSensor) -> Data Type Conversion27/1
  LegMedulla_2L/2(MotorEncoder) -> Data Type Conversion26/1
  LegMedulla_2L/1(LegEncoder) -> Data Type Conversion25/1
  LegMedulla_1L/23(KneeForce1) -> Data Type Conversion23/1
  LegMedulla_1L/22(Amp2MeasuredCurrent) -> Data Type Conversion22/1
  LegMedulla_1L/21(Amp1MeasuredCurrent) -> Data Type Conversion21/1
  LegMedulla_1L/20(Thermistor5) -> Data Type Conversion20/1
  LegMedulla_1L/19(Thermistor4) -> Data Type Conversion19/1
  LegMedulla_1L/18(Thermistor3) -> Data Type Conversion18/1
  LegMedulla_1L/17(Thermistor2) -> Data Type Conversion17/1
  LegMedulla_1L/16(Thermistor1) -> Data Type Conversion16/1
  LegMedulla_1L/15(Thermistor0) -> Data Type Conversion15/1
  LegMedulla_1L/14(LogicVoltage) -> Data Type Conversion14/1
  LegMedulla_1L/13(MotorVoltage) -> Data Type Conversion13/1
  LegMedulla_1L/12(IncEncoderTimestamp) -> Data Type Conversion12/1
  LegMedulla_1L/11(MotorEncoderTimestamp) -> Data Type Conversion11/1
  LegMedulla_1L/10(LegEncoderTimestamp) -> Data Type Conversion10/1
  LegMedulla_1L/9(IncEncoder) -> Data Type Conversion9/1
  LegMedulla_1L/8(ErrorFlags) -> Data Type Conversion8/1
  LegMedulla_1L/7(Counter) -> Data Type Conversion7/1
  LegMedulla_1L/6(State) -> Data Type Conversion6/1
  LegMedulla_1L/5(ID) -> Data Type Conversion5/1
  LegMedulla_1L/4(LimitSwitch) -> Data Type Conversion4/1
  LegMedulla_1L/3(ToeSensor) -> Data Type Conversion2/1
  LegMedulla_1L/2(MotorEncoder) -> Data Type Conversion1/1
  EncodeSwitches/1(LimitSwitchesEncoded) -> LimitSwitches/1
  Mux11/1 -> ToeSwitches/1
  EtherCAT Init/1 -> Data Type Conversion97/1
  BoomMedulla/2(Z_Encoder) -> Data Type Conversion140/1
  BoomMedulla/1(OSU_X_Encoder) -> Data Type Conversion141/1
  [Reset] -> convert_mtr_current_to_pwm/3(Reset)
  Data Type Conversion97/1 -> [EtherCATStatus]
  [EtherCATStatus] -> EtherCATStatus/1
  [EtherCATStatus] -> Reset/2(EtherCATStatus)

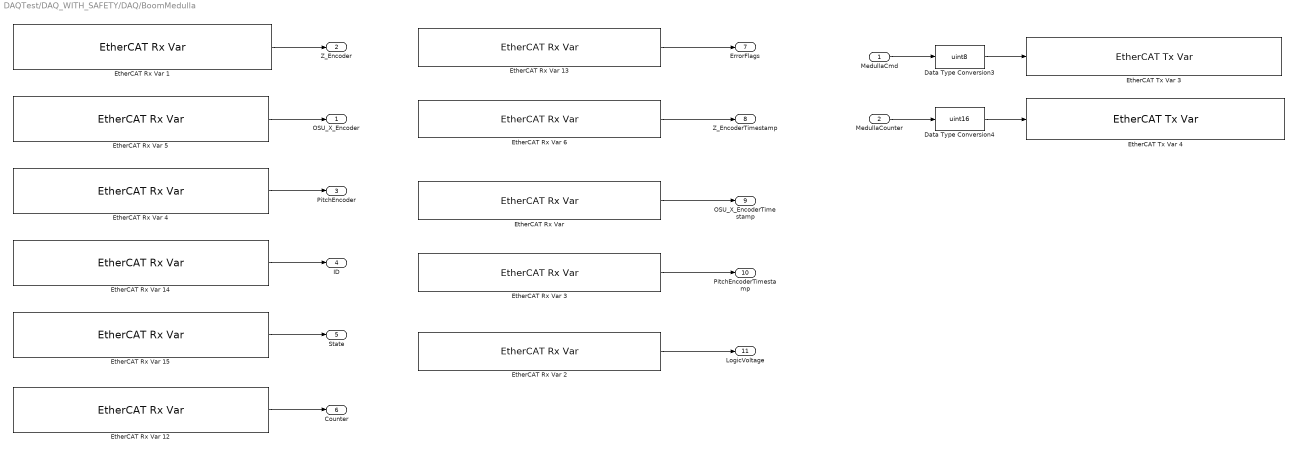
== system DAQTest/DAQ_WITH_SAFETY/DAQ/BoomMedulla ==
  MedullaCmd : Inport
  MedullaCounter : Inport  Port=2
  Data Type Conversion3 : DataTypeConversion  OutDataTypeStr=uint8
  Data Type Conversion4 : DataTypeConversion  OutDataTypeStr=uint16
  "EtherCAT Rx Var " : xpcethercatlib/EtherCAT Rx Var   Priority=2  sig_name=Box 7 (ATRIAS 2.1 Boom (Medulla 1.5)).X Encoder.Timestamp  sig_offset=2464  sig_type=uint16  type_size=16  sig_dim=1  device_id=0  sample_time=0.001000
  EtherCAT Rx Var 1 : xpcethercatlib/EtherCAT Rx Var   Priority=2  sig_name=Box 7 (ATRIAS 2.1 Boom (Medulla 1.5)).Z Encoder.Encoder  sig_offset=2528  sig_type=uint32  type_size=32  sig_dim=1  device_id=0  sample_time=0.001000
  EtherCAT Rx Var 12 : xpcethercatlib/EtherCAT Rx Var   Priority=2  sig_name=Box 7 (ATRIAS 2.1 Boom (Medulla 1.5)).uController Status.Counter  sig_offset=2416  sig_type=uint8  type_size=8  sig_dim=1  device_id=0  sample_time=0.001000
  EtherCAT Rx Var 13 : xpcethercatlib/EtherCAT Rx Var   Priority=2  sig_name=Box 7 (ATRIAS 2.1 Boom (Medulla 1.5)).uController Status.Error Flags  sig_offset=2424  sig_type=uint8  type_size=8  sig_dim=1  device_id=0  sample_time=0.001000
  EtherCAT Rx Var 14 : xpcethercatlib/EtherCAT Rx Var   Priority=2  sig_name=Box 7 (ATRIAS 2.1 Boom (Medulla 1.5)).uController Status.ID  sig_offset=2400  sig_type=uint8  type_size=8  sig_dim=1  device_id=0  sample_time=0.001000
  EtherCAT Rx Var 15 : xpcethercatlib/EtherCAT Rx Var   Priority=2  sig_name=Box 7 (ATRIAS 2.1 Boom (Medulla 1.5)).uController Status.State  sig_offset=2408  sig_type=uint8  type_size=8  sig_dim=1  device_id=0  sample_time=0.001000
  EtherCAT Rx Var 2 : xpcethercatlib/EtherCAT Rx Var   Priority=2  sig_name=Box 7 (ATRIAS 2.1 Boom (Medulla 1.5)).Power.Logic Voltage  sig_offset=2576  sig_type=uint16  type_size=16  sig_dim=1  device_id=0  sample_time=0.001000
  EtherCAT Rx Var 3 : xpcethercatlib/EtherCAT Rx Var   Priority=2  sig_name=Box 7 (ATRIAS 2.1 Boom (Medulla 1.5)).Pitch Encoder.Timestamp  sig_offset=2512  sig_type=uint16  type_size=16  sig_dim=1  device_id=0  sample_time=0.001000
  EtherCAT Rx Var 4 : xpcethercatlib/EtherCAT Rx Var   Priority=2  sig_name=Box 7 (ATRIAS 2.1 Boom (Medulla 1.5)).Pitch Encoder.Encoder  sig_offset=2480  sig_type=uint32  type_size=32  sig_dim=1  device_id=0  sample_time=0.001000
  EtherCAT Rx Var 5 : xpcethercatlib/EtherCAT Rx Var   Priority=2  sig_name=Box 7 (ATRIAS 2.1 Boom (Medulla 1.5)).X Encoder.Encoder  sig_offset=2432  sig_type=uint32  type_size=32  sig_dim=1  device_id=0  sample_time=0.001000
  EtherCAT Rx Var 6 : xpcethercatlib/EtherCAT Rx Var   Priority=2  sig_name=Box 7 (ATRIAS 2.1 Boom (Medulla 1.5)).Z Encoder.Timestamp  sig_offset=2560  sig_type=uint16  type_size=16  sig_dim=1  device_id=0  sample_time=0.001000
  EtherCAT Tx Var 3 : xpcethercatlib/EtherCAT Tx Var   Priority=3  sig_name=Box 7 (ATRIAS 2.1 Boom (Medulla 1.5)).uControllerInput.Command  sig_offset=2400  sig_type=uint8  type_size=8  sig_dim=1  device_id=0  sample_time=0.001000
  EtherCAT Tx Var 4 : xpcethercatlib/EtherCAT Tx Var   Priority=3  sig_name=Box 7 (ATRIAS 2.1 Boom (Medulla 1.5)).uControllerInput.Counter  sig_offset=2408  sig_type=uint16  type_size=16  sig_dim=1  device_id=0  sample_time=0.001000
  OSU_X_Encoder : Outport
  Z_Encoder : Outport  Port=2
  PitchEncoder : Outport  Port=3
  ID : Outport  Port=4
  State : Outport  Port=5
  Counter : Outport  Port=6
  ErrorFlags : Outport  Port=7
  Z_EncoderTimestamp : Outport  Port=8
  OSU_X_EncoderTimestamp : Outport  Port=9
  PitchEncoderTimestamp : Outport  Port=10
  LogicVoltage : Outport  Port=11
  wires:
  EtherCAT Rx Var 2/1 -> LogicVoltage/1
  EtherCAT Rx Var 3/1 -> PitchEncoderTimestamp/1
  "EtherCAT Rx Var "/1 -> OSU_X_EncoderTimestamp/1
  EtherCAT Rx Var 6/1 -> Z_EncoderTimestamp/1
  EtherCAT Rx Var 13/1 -> ErrorFlags/1
  EtherCAT Rx Var 12/1 -> Counter/1
  EtherCAT Rx Var 15/1 -> State/1
  EtherCAT Rx Var 14/1 -> ID/1
  EtherCAT Rx Var 4/1 -> PitchEncoder/1
  EtherCAT Rx Var 5/1 -> OSU_X_Encoder/1
  EtherCAT Rx Var 1/1 -> Z_Encoder/1
  MedullaCounter/1 -> Data Type Conversion4/1
  MedullaCmd/1 -> Data Type Conversion3/1
  Data Type Conversion4/1 -> EtherCAT Tx Var 4/1
  Data Type Conversion3/1 -> EtherCAT Tx Var 3/1

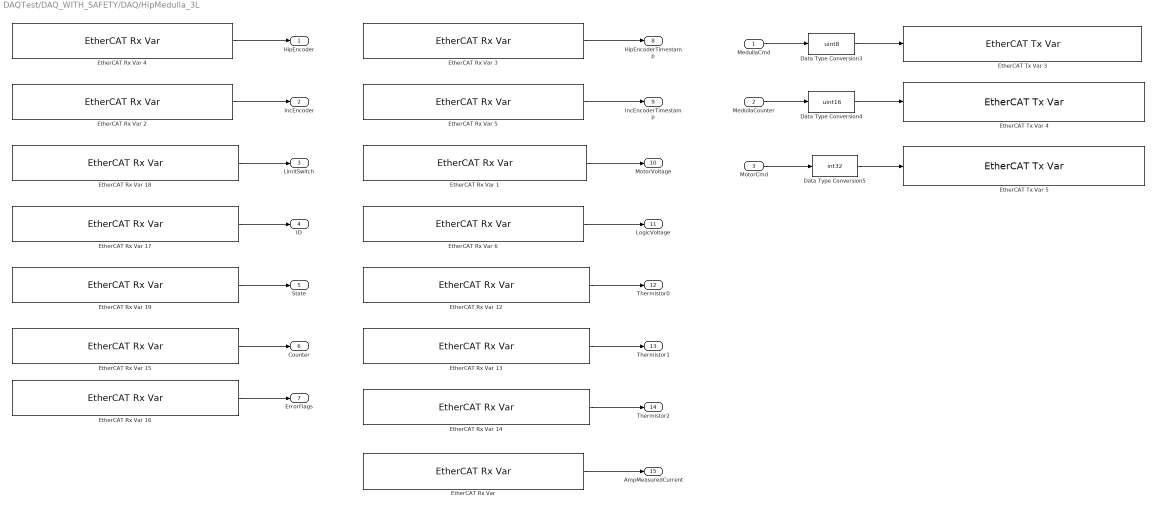
== system DAQTest/DAQ_WITH_SAFETY/DAQ/HipMedulla_3L ==
  MedullaCmd : Inport
  MedullaCounter : Inport  Port=2
  MotorCmd : Inport  Port=3
  Data Type Conversion3 : DataTypeConversion  OutDataTypeStr=uint8
  Data Type Conversion4 : DataTypeConversion  OutDataTypeStr=uint16
  Data Type Conversion5 : DataTypeConversion  OutDataTypeStr=int32
  "EtherCAT Rx Var " : xpcethercatlib/EtherCAT Rx Var   Priority=2  sig_name=Box 6 (ATRIAS 2.1 Hip (Medulla 1.5)).Measured Current.Amp Measured Current  sig_offset=2352  sig_type=int16  type_size=16  sig_dim=1  device_id=0  sample_time=0.001000
  EtherCAT Rx Var 1 : xpcethercatlib/EtherCAT Rx Var   Priority=2  sig_name=Box 6 (ATRIAS 2.1 Hip (Medulla 1.5)).Power.Motor Voltage  sig_offset=2272  sig_type=uint16  type_size=16  sig_dim=1  device_id=0  sample_time=0.001000
  EtherCAT Rx Var 12 : xpcethercatlib/EtherCAT Rx Var   Priority=2  sig_name=Box 6 (ATRIAS 2.1 Hip (Medulla 1.5)).Thermistors.Thermistor 0  sig_offset=2304  sig_type=uint16  type_size=16  sig_dim=1  device_id=0  sample_time=0.001000
  EtherCAT Rx Var 13 : xpcethercatlib/EtherCAT Rx Var   Priority=2  sig_name=Box 6 (ATRIAS 2.1 Hip (Medulla 1.5)).Thermistors.Thermistor 1  sig_offset=2320  sig_type=uint16  type_size=16  sig_dim=1  device_id=0  sample_time=0.001000
  EtherCAT Rx Var 14 : xpcethercatlib/EtherCAT Rx Var   Priority=2  sig_name=Box 6 (ATRIAS 2.1 Hip (Medulla 1.5)).Thermistors.Thermistor 2  sig_offset=2336  sig_type=uint16  type_size=16  sig_dim=1  device_id=0  sample_time=0.001000
  EtherCAT Rx Var 15 : xpcethercatlib/EtherCAT Rx Var   Priority=2  sig_name=Box 6 (ATRIAS 2.1 Hip (Medulla 1.5)).uController Status.Counter  sig_offset=2200  sig_type=uint8  type_size=8  sig_dim=1  device_id=0  sample_time=0.001000
  EtherCAT Rx Var 16 : xpcethercatlib/EtherCAT Rx Var   Priority=2  sig_name=Box 6 (ATRIAS 2.1 Hip (Medulla 1.5)).uController Status.Error Flags  sig_offset=2208  sig_type=uint8  type_size=8  sig_dim=1  device_id=0  sample_time=0.001000
  EtherCAT Rx Var 17 : xpcethercatlib/EtherCAT Rx Var   Priority=2  sig_name=Box 6 (ATRIAS 2.1 Hip (Medulla 1.5)).uController Status.ID  sig_offset=2184  sig_type=uint8  type_size=8  sig_dim=1  device_id=0  sample_time=0.001000
  EtherCAT Rx Var 18 : xpcethercatlib/EtherCAT Rx Var   Priority=2  sig_name=Box 6 (ATRIAS 2.1 Hip (Medulla 1.5)).uController Status.Limit Switch  sig_offset=2216  sig_type=uint8  type_size=8  sig_dim=1  device_id=0  sample_time=0.001000
  EtherCAT Rx Var 19 : xpcethercatlib/EtherCAT Rx Var   Priority=2  sig_name=Box 6 (ATRIAS 2.1 Hip (Medulla 1.5)).uController Status.State  sig_offset=2192  sig_type=uint8  type_size=8  sig_dim=1  device_id=0  sample_time=0.001000
  EtherCAT Rx Var 2 : xpcethercatlib/EtherCAT Rx Var   Priority=2  sig_name=Box 6 (ATRIAS 2.1 Hip (Medulla 1.5)).Incremental Encoder.Incremental Encoder  sig_offset=2368  sig_type=uint16  type_size=16  sig_dim=1  device_id=0  sample_time=0.001000
  EtherCAT Rx Var 3 : xpcethercatlib/EtherCAT Rx Var   Priority=2  sig_name=Box 6 (ATRIAS 2.1 Hip (Medulla 1.5)).Hip Encoder.Timestamp  sig_offset=2256  sig_type=uint16  type_size=16  sig_dim=1  device_id=0  sample_time=0.001000
  EtherCAT Rx Var 4 : xpcethercatlib/EtherCAT Rx Var   Priority=2  sig_name=Box 6 (ATRIAS 2.1 Hip (Medulla 1.5)).Hip Encoder.Encoder  sig_offset=2224  sig_type=uint32  type_size=32  sig_dim=1  device_id=0  sample_time=0.001000
  EtherCAT Rx Var 5 : xpcethercatlib/EtherCAT Rx Var   Priority=2  sig_name=Box 6 (ATRIAS 2.1 Hip (Medulla 1.5)).Incremental Encoder.Incremental Encoder Timestamp  sig_offset=2384  sig_type=uint16  type_size=16  sig_dim=1  device_id=0  sample_time=0.001000
  EtherCAT Rx Var 6 : xpcethercatlib/EtherCAT Rx Var   Priority=2  sig_name=Box 6 (ATRIAS 2.1 Hip (Medulla 1.5)).Power.Logic Voltage  sig_offset=2288  sig_type=uint16  type_size=16  sig_dim=1  device_id=0  sample_time=0.001000
  EtherCAT Tx Var 3 : xpcethercatlib/EtherCAT Tx Var   Priority=3  sig_name=Box 6 (ATRIAS 2.1 Hip (Medulla 1.5)).uControllerInput.Command  sig_offset=2184  sig_type=uint8  type_size=8  sig_dim=1  device_id=0  sample_time=0.001000
  EtherCAT Tx Var 4 : xpcethercatlib/EtherCAT Tx Var   Priority=3  sig_name=Box 6 (ATRIAS 2.1 Hip (Medulla 1.5)).uControllerInput.Counter  sig_offset=2192  sig_type=uint16  type_size=16  sig_dim=1  device_id=0  sample_time=0.001000
  EtherCAT Tx Var 5 : xpcethercatlib/EtherCAT Tx Var   Priority=3  sig_name=Box 6 (ATRIAS 2.1 Hip (Medulla 1.5)).uControllerInput.Motor Current  sig_offset=2208  sig_type=int32  type_size=32  sig_dim=1  device_id=0  sample_time=0.001000
  HipEncoder : Outport
  IncEncoder : Outport  Port=2
  LimitSwitch : Outport  Port=3
  ID : Outport  Port=4
  State : Outport  Port=5
  Counter : Outport  Port=6
  ErrorFlags : Outport  Port=7
  HipEncoderTimestamp : Outport  Port=8
  IncEncoderTimestamp : Outport  Port=9
  MotorVoltage : Outport  Port=10
  LogicVoltage : Outport  Port=11
  Thermistor0 : Outport  Port=12
  Thermistor1 : Outport  Port=13
  Thermistor2 : Outport  Port=14
  AmpMeasuredCurrent : Outport  Port=15
  wires:
  "EtherCAT Rx Var "/1 -> AmpMeasuredCurrent/1
  EtherCAT Rx Var 14/1 -> Thermistor2/1
  EtherCAT Rx Var 13/1 -> Thermistor1/1
  EtherCAT Rx Var 12/1 -> Thermistor0/1
  EtherCAT Rx Var 1/1 -> MotorVoltage/1
  EtherCAT Rx Var 6/1 -> LogicVoltage/1
  EtherCAT Rx Var 16/1 -> ErrorFlags/1
  EtherCAT Rx Var 19/1 -> State/1
  EtherCAT Rx Var 18/1 -> LimitSwitch/1
  EtherCAT Rx Var 17/1 -> ID/1
  EtherCAT Rx Var 15/1 -> Counter/1
  EtherCAT Rx Var 2/1 -> IncEncoder/1
  EtherCAT Rx Var 3/1 -> HipEncoderTimestamp/1
  EtherCAT Rx Var 4/1 -> HipEncoder/1
  EtherCAT Rx Var 5/1 -> IncEncoderTimestamp/1
  MotorCmd/1 -> Data Type Conversion5/1
  MedullaCounter/1 -> Data Type Conversion4/1
  MedullaCmd/1 -> Data Type Conversion3/1
  Data Type Conversion5/1 -> EtherCAT Tx Var 5/1
  Data Type Conversion4/1 -> EtherCAT Tx Var 4/1
  Data Type Conversion3/1 -> EtherCAT Tx Var 3/1
